simulink model "EPT"  (R2019b)
settings: Solver=FixedStepDiscrete  StartTime=0.0  StopTime=5  FixedStep=0.005  RelTol=1e-3  EnableMultiTasking=on
PreLoadFcn:
  | try, model_open; catch, disp('Error occurred while executing model pre-load callback: model_open.m'); disp('Please assure that the MATLAB working directory is set to the model directory before opening.'); end
InitFcn:
  | try, model_open; catch, end
undefined symbols (not defined in the file or in its folder): Bridge, GCM, H, ln, raptor_get_param_eval, raptor_get_safe_string, raptor_xcp_function
libraries: Raptor_lib x2810, simulink x374, hdlsllib x19
(part 10 of 45)

== system EPT/Foreground_TimeBase_5ms/Oil//Water//Pack Cooling System/AirC1/Delay1 ==
  Condition : Inport
  TimeCount : Inport  Port=2
  Constant10 : Constant
  Constant11 : Constant  Value=0
  Constant8 : Constant  Value=0
  CycleTrigger : Subsystem
  Switch2 : Switch  Threshold=1
  Switch3 : Switch  Threshold=1
  Unit Delay1 : UnitDelay  SampleTime=-1  HasFrameUpgradeWarning=on
  Unit Delay3 : UnitDelay  SampleTime=-1  HasFrameUpgradeWarning=on
  Output : Outport  VectorParamsAs1DForOutWhenUnconnected=off
  wires:
  TimeCount/1 -> CycleTrigger/2(In2)
  Condition/1 -> Switch3/2
  Constant8/1 -> Switch2/1
  CycleTrigger/1(Trigger) -> Switch2/2, Unit Delay3/1
  Constant10/1 -> Switch2/3
  Switch3/1 -> CycleTrigger/1(In1)
  Switch2/1 -> Unit Delay1/1
  Constant11/1 -> Switch3/3
  Unit Delay1/1 -> Switch3/1
  Unit Delay3/1 -> Output/1

== system EPT/Foreground_TimeBase_5ms/Oil//Water//Pack Cooling System/AirC1/Delay2 ==
  Condition : Inport
  TimeCount : Inport  Port=2
  Constant10 : Constant
  Constant11 : Constant  Value=0
  Constant8 : Constant  Value=0
  CycleTrigger : Subsystem
  Switch2 : Switch  Threshold=1
  Switch3 : Switch  Threshold=1
  Unit Delay1 : UnitDelay  SampleTime=-1  HasFrameUpgradeWarning=on
  Unit Delay3 : UnitDelay  SampleTime=-1  HasFrameUpgradeWarning=on
  Output : Outport  VectorParamsAs1DForOutWhenUnconnected=off
  wires:
  TimeCount/1 -> CycleTrigger/2(In2)
  Condition/1 -> Switch3/2
  Constant8/1 -> Switch2/1
  CycleTrigger/1(Trigger) -> Switch2/2, Unit Delay3/1
  Constant10/1 -> Switch2/3
  Switch3/1 -> CycleTrigger/1(In1)
  Switch2/1 -> Unit Delay1/1
  Constant11/1 -> Switch3/3
  Unit Delay1/1 -> Switch3/1
  Unit Delay3/1 -> Output/1

== system EPT/Foreground_TimeBase_5ms/Oil//Water//Pack Cooling System/AirC1/Delay3 ==
  Condition : Inport
  TimeCount : Inport  Port=2
  Constant10 : Constant
  Constant11 : Constant  Value=0
  Constant8 : Constant  Value=0
  CycleTrigger : Subsystem
  Switch2 : Switch  Threshold=1
  Switch3 : Switch  Threshold=1
  Unit Delay1 : UnitDelay  SampleTime=-1  HasFrameUpgradeWarning=on
  Unit Delay3 : UnitDelay  SampleTime=-1  HasFrameUpgradeWarning=on
  Output : Outport  VectorParamsAs1DForOutWhenUnconnected=off
  wires:
  Unit Delay3/1 -> Output/1
  Unit Delay1/1 -> Switch3/1
  Constant11/1 -> Switch3/3
  Switch2/1 -> Unit Delay1/1
  Switch3/1 -> CycleTrigger/1(In1)
  Constant10/1 -> Switch2/3
  CycleTrigger/1(Trigger) -> Unit Delay3/1, Switch2/2
  Constant8/1 -> Switch2/1
  Condition/1 -> Switch3/2
  TimeCount/1 -> CycleTrigger/2(In2)

== system EPT/Foreground_TimeBase_5ms/Oil//Water//Pack Cooling System/AirC1/Delay5 ==
  Condition : Inport
  TimeCount : Inport  Port=2
  Constant10 : Constant
  Constant11 : Constant  Value=0
  Constant8 : Constant  Value=0
  CycleTrigger : Subsystem
  Switch2 : Switch  Threshold=1
  Switch3 : Switch  Threshold=1
  Unit Delay1 : UnitDelay  SampleTime=-1  HasFrameUpgradeWarning=on
  Unit Delay3 : UnitDelay  SampleTime=-1  HasFrameUpgradeWarning=on
  Output : Outport  VectorParamsAs1DForOutWhenUnconnected=off
  wires:
  Unit Delay3/1 -> Output/1
  Unit Delay1/1 -> Switch3/1
  Constant11/1 -> Switch3/3
  Switch2/1 -> Unit Delay1/1
  Switch3/1 -> CycleTrigger/1(In1)
  Constant10/1 -> Switch2/3
  CycleTrigger/1(Trigger) -> Unit Delay3/1, Switch2/2
  Constant8/1 -> Switch2/1
  Condition/1 -> Switch3/2
  TimeCount/1 -> CycleTrigger/2(In2)

== system EPT/Foreground_TimeBase_5ms/Oil//Water//Pack Cooling System/AirC1/Delay6 ==
  Condition : Inport
  TimeCount : Inport  Port=2
  Constant10 : Constant
  Constant11 : Constant  Value=0
  Constant8 : Constant  Value=0
  CycleTrigger : Subsystem
  Switch2 : Switch  Threshold=1
  Switch3 : Switch  Threshold=1
  Unit Delay1 : UnitDelay  SampleTime=-1  HasFrameUpgradeWarning=on
  Unit Delay3 : UnitDelay  SampleTime=-1  HasFrameUpgradeWarning=on
  Output : Outport  VectorParamsAs1DForOutWhenUnconnected=off
  wires:
  Unit Delay3/1 -> Output/1
  Unit Delay1/1 -> Switch3/1
  Constant11/1 -> Switch3/3
  Switch2/1 -> Unit Delay1/1
  Switch3/1 -> CycleTrigger/1(In1)
  Constant10/1 -> Switch2/3
  CycleTrigger/1(Trigger) -> Unit Delay3/1, Switch2/2
  Constant8/1 -> Switch2/1
  Condition/1 -> Switch3/2
  TimeCount/1 -> CycleTrigger/2(In2)

== system EPT/Foreground_TimeBase_5ms/Oil//Water//Pack Cooling System/AirC1/Delay7 ==
  Condition : Inport
  TimeCount : Inport  Port=2
  Constant10 : Constant
  Constant11 : Constant  Value=0
  Constant8 : Constant  Value=0
  CycleTrigger : Subsystem
  Switch2 : Switch  Threshold=1
  Switch3 : Switch  Threshold=1
  Unit Delay1 : UnitDelay  SampleTime=-1  HasFrameUpgradeWarning=on
  Unit Delay3 : UnitDelay  SampleTime=-1  HasFrameUpgradeWarning=on
  Output : Outport  VectorParamsAs1DForOutWhenUnconnected=off
  wires:
  Unit Delay3/1 -> Output/1
  Unit Delay1/1 -> Switch3/1
  Constant11/1 -> Switch3/3
  Switch2/1 -> Unit Delay1/1
  Switch3/1 -> CycleTrigger/1(In1)
  Constant10/1 -> Switch2/3
  CycleTrigger/1(Trigger) -> Unit Delay3/1, Switch2/2
  Constant8/1 -> Switch2/1
  Condition/1 -> Switch3/2
  TimeCount/1 -> CycleTrigger/2(In2)

== system EPT/Foreground_TimeBase_5ms/Oil//Water//Pack Cooling System/AirC1/Latch ==
  Latch : Inport
  Reset : Inport  Port=2
  Switch1 : Switch  Criteria=u2 > Threshold
  Switch3 : Switch  Criteria=u2 > Threshold
  Unit Delay1 : UnitDelay  SampleTime=-1  HasFrameUpgradeWarning=on
  Output : Outport  VectorParamsAs1DForOutWhenUnconnected=off
  wires:
  Unit Delay1/1 -> Switch1/3
  Switch3/1 -> Output/1, Unit Delay1/1
  Reset/1 -> Switch3/2
  Latch/1 -> Switch1/1, Switch1/2
  Switch1/1 -> Switch3/3

== system EPT/Foreground_TimeBase_5ms/Oil//Water//Pack Cooling System/AirC1/Latch1 ==
  Latch : Inport
  Reset : Inport  Port=2
  Switch1 : Switch  Criteria=u2 > Threshold
  Switch3 : Switch  Criteria=u2 > Threshold
  Unit Delay1 : UnitDelay  SampleTime=-1  HasFrameUpgradeWarning=on
  Output : Outport  VectorParamsAs1DForOutWhenUnconnected=off
  wires:
  Unit Delay1/1 -> Switch1/3
  Switch3/1 -> Output/1, Unit Delay1/1
  Reset/1 -> Switch3/2
  Latch/1 -> Switch1/1, Switch1/2
  Switch1/1 -> Switch3/3

== system EPT/Foreground_TimeBase_5ms/Oil//Water//Pack Cooling System/AirC1/Latch2 ==
  Latch : Inport
  Reset : Inport  Port=2
  Switch1 : Switch  Criteria=u2 > Threshold
  Switch3 : Switch  Criteria=u2 > Threshold
  Unit Delay1 : UnitDelay  SampleTime=-1  HasFrameUpgradeWarning=on
  Output : Outport  VectorParamsAs1DForOutWhenUnconnected=off
  wires:
  Switch1/1 -> Switch3/3
  Latch/1 -> Switch1/2, Switch1/1
  Reset/1 -> Switch3/2
  Switch3/1 -> Unit Delay1/1, Output/1
  Unit Delay1/1 -> Switch1/3

== system EPT/Foreground_TimeBase_5ms/Oil//Water//Pack Cooling System/Delay1/CycleTrigger ==
  In1 : Inport
  In2 : Inport  Port=2
  Add : Sum
  Add1 : Sum
  Add2 : Sum  Inputs=+-
  Constant1 : Constant
  Constant2 : Constant  Value=0
  Constant3 : Constant
  Data Type Conversion1 : DataTypeConversion
  Data Type Conversion2 : DataTypeConversion
  Display : Display
  Relational Operator1 : RelationalOperator  OutDataTypeStr=boolean  RndMeth=Simplest
  Saturation : Saturate  UpperLimit=inf  LowerLimit=2
  Scope : Scope
  Scope1 : Scope
  Scope2 : Scope
  Switch : Switch  Threshold=1
  Unit Delay : UnitDelay  SampleTime=-1  HasFrameUpgradeWarning=on
  Unit Delay1 : UnitDelay  SampleTime=-1  HasFrameUpgradeWarning=on
  Trigger : Outport  VectorParamsAs1DForOutWhenUnconnected=off
  wires:
  Saturation/1 -> Add2/1
  Add/1 -> Switch/1
  In1/1 -> Data Type Conversion2/1
  Unit Delay/1 -> Add/1
  Switch/1 -> Relational Operator1/1, Scope1/1, Unit Delay/1
  Add1/1 -> Scope/1, Unit Delay1/1, Display/1
  Unit Delay1/1 -> Add1/1
  Constant1/1 -> Add1/2
  Relational Operator1/1 -> Scope2/1, Trigger/1
  Data Type Conversion1/1 -> Relational Operator1/2
  Constant2/1 -> Switch/3
  Data Type Conversion2/1 -> Add/2, Switch/2
  Add2/1 -> Data Type Conversion1/1
  In2/1 -> Saturation/1
  Constant3/1 -> Add2/2

== system EPT/Foreground_TimeBase_5ms/Oil//Water//Pack Cooling System/Delay2/CycleTrigger ==
  In1 : Inport
  In2 : Inport  Port=2
  Add : Sum
  Add1 : Sum
  Add2 : Sum  Inputs=+-
  Constant1 : Constant
  Constant2 : Constant  Value=0
  Constant3 : Constant
  Data Type Conversion1 : DataTypeConversion
  Data Type Conversion2 : DataTypeConversion
  Display : Display
  Relational Operator1 : RelationalOperator  OutDataTypeStr=boolean  RndMeth=Simplest
  Saturation : Saturate  UpperLimit=inf  LowerLimit=2
  Scope : Scope
  Scope1 : Scope
  Scope2 : Scope
  Switch : Switch  Threshold=1
  Unit Delay : UnitDelay  SampleTime=-1  HasFrameUpgradeWarning=on
  Unit Delay1 : UnitDelay  SampleTime=-1  HasFrameUpgradeWarning=on
  Trigger : Outport  VectorParamsAs1DForOutWhenUnconnected=off
  wires:
  Saturation/1 -> Add2/1
  Add/1 -> Switch/1
  In1/1 -> Data Type Conversion2/1
  Unit Delay/1 -> Add/1
  Switch/1 -> Relational Operator1/1, Scope1/1, Unit Delay/1
  Add1/1 -> Scope/1, Unit Delay1/1, Display/1
  Unit Delay1/1 -> Add1/1
  Constant1/1 -> Add1/2
  Relational Operator1/1 -> Scope2/1, Trigger/1
  Data Type Conversion1/1 -> Relational Operator1/2
  Constant2/1 -> Switch/3
  Data Type Conversion2/1 -> Add/2, Switch/2
  Add2/1 -> Data Type Conversion1/1
  In2/1 -> Saturation/1
  Constant3/1 -> Add2/2

== system EPT/Foreground_TimeBase_5ms/Oil//Water//Pack Cooling System/Delay3/CycleTrigger ==
  In1 : Inport
  In2 : Inport  Port=2
  Add : Sum
  Add1 : Sum
  Add2 : Sum  Inputs=+-
  Constant1 : Constant
  Constant2 : Constant  Value=0
  Constant3 : Constant
  Data Type Conversion1 : DataTypeConversion
  Data Type Conversion2 : DataTypeConversion
  Display : Display
  Relational Operator1 : RelationalOperator  OutDataTypeStr=boolean  RndMeth=Simplest
  Saturation : Saturate  UpperLimit=inf  LowerLimit=2
  Scope : Scope
  Scope1 : Scope
  Scope2 : Scope
  Switch : Switch  Threshold=1
  Unit Delay : UnitDelay  SampleTime=-1  HasFrameUpgradeWarning=on
  Unit Delay1 : UnitDelay  SampleTime=-1  HasFrameUpgradeWarning=on
  Trigger : Outport  VectorParamsAs1DForOutWhenUnconnected=off
  wires:
  Constant3/1 -> Add2/2
  In2/1 -> Saturation/1
  Add2/1 -> Data Type Conversion1/1
  Data Type Conversion2/1 -> Switch/2, Add/2
  Constant2/1 -> Switch/3
  Data Type Conversion1/1 -> Relational Operator1/2
  Relational Operator1/1 -> Trigger/1, Scope2/1
  Constant1/1 -> Add1/2
  Unit Delay1/1 -> Add1/1
  Add1/1 -> Display/1, Unit Delay1/1, Scope/1
  Switch/1 -> Unit Delay/1, Scope1/1, Relational Operator1/1
  Unit Delay/1 -> Add/1
  In1/1 -> Data Type Conversion2/1
  Add/1 -> Switch/1
  Saturation/1 -> Add2/1

== system EPT/Foreground_TimeBase_5ms/Oil//Water//Pack Cooling System/Delay5/CycleTrigger ==
  In1 : Inport
  In2 : Inport  Port=2
  Add : Sum
  Add1 : Sum
  Add2 : Sum  Inputs=+-
  Constant1 : Constant
  Constant2 : Constant  Value=0
  Constant3 : Constant
  Data Type Conversion1 : DataTypeConversion
  Data Type Conversion2 : DataTypeConversion
  Display : Display
  Relational Operator1 : RelationalOperator  OutDataTypeStr=boolean  RndMeth=Simplest
  Saturation : Saturate  UpperLimit=inf  LowerLimit=2
  Scope : Scope
  Scope1 : Scope
  Scope2 : Scope
  Switch : Switch  Threshold=1
  Unit Delay : UnitDelay  SampleTime=-1  HasFrameUpgradeWarning=on
  Unit Delay1 : UnitDelay  SampleTime=-1  HasFrameUpgradeWarning=on
  Trigger : Outport  VectorParamsAs1DForOutWhenUnconnected=off
  wires:
  Constant3/1 -> Add2/2
  In2/1 -> Saturation/1
  Add2/1 -> Data Type Conversion1/1
  Data Type Conversion2/1 -> Switch/2, Add/2
  Constant2/1 -> Switch/3
  Data Type Conversion1/1 -> Relational Operator1/2
  Relational Operator1/1 -> Trigger/1, Scope2/1
  Constant1/1 -> Add1/2
  Unit Delay1/1 -> Add1/1
  Add1/1 -> Display/1, Unit Delay1/1, Scope/1
  Switch/1 -> Unit Delay/1, Scope1/1, Relational Operator1/1
  Unit Delay/1 -> Add/1
  In1/1 -> Data Type Conversion2/1
  Add/1 -> Switch/1
  Saturation/1 -> Add2/1

== system EPT/Foreground_TimeBase_5ms/Oil//Water//Pack Cooling System/Delay6/CycleTrigger ==
  In1 : Inport
  In2 : Inport  Port=2
  Add : Sum
  Add1 : Sum
  Add2 : Sum  Inputs=+-
  Constant1 : Constant
  Constant2 : Constant  Value=0
  Constant3 : Constant
  Data Type Conversion1 : DataTypeConversion
  Data Type Conversion2 : DataTypeConversion
  Display : Display
  Relational Operator1 : RelationalOperator  OutDataTypeStr=boolean  RndMeth=Simplest
  Saturation : Saturate  UpperLimit=inf  LowerLimit=2
  Scope : Scope
  Scope1 : Scope
  Scope2 : Scope
  Switch : Switch  Threshold=1
  Unit Delay : UnitDelay  SampleTime=-1  HasFrameUpgradeWarning=on
  Unit Delay1 : UnitDelay  SampleTime=-1  HasFrameUpgradeWarning=on
  Trigger : Outport  VectorParamsAs1DForOutWhenUnconnected=off
  wires:
  Constant3/1 -> Add2/2
  In2/1 -> Saturation/1
  Add2/1 -> Data Type Conversion1/1
  Data Type Conversion2/1 -> Switch/2, Add/2
  Constant2/1 -> Switch/3
  Data Type Conversion1/1 -> Relational Operator1/2
  Relational Operator1/1 -> Trigger/1, Scope2/1
  Constant1/1 -> Add1/2
  Unit Delay1/1 -> Add1/1
  Add1/1 -> Display/1, Unit Delay1/1, Scope/1
  Switch/1 -> Unit Delay/1, Scope1/1, Relational Operator1/1
  Unit Delay/1 -> Add/1
  In1/1 -> Data Type Conversion2/1
  Add/1 -> Switch/1
  Saturation/1 -> Add2/1

== system EPT/Foreground_TimeBase_5ms/Oil//Water//Pack Cooling System/Delay7/CycleTrigger ==
  In1 : Inport
  In2 : Inport  Port=2
  Add : Sum
  Add1 : Sum
  Add2 : Sum  Inputs=+-
  Constant1 : Constant
  Constant2 : Constant  Value=0
  Constant3 : Constant
  Data Type Conversion1 : DataTypeConversion
  Data Type Conversion2 : DataTypeConversion
  Display : Display
  Relational Operator1 : RelationalOperator  OutDataTypeStr=boolean  RndMeth=Simplest
  Saturation : Saturate  UpperLimit=inf  LowerLimit=2
  Scope : Scope
  Scope1 : Scope
  Scope2 : Scope
  Switch : Switch  Threshold=1
  Unit Delay : UnitDelay  SampleTime=-1  HasFrameUpgradeWarning=on
  Unit Delay1 : UnitDelay  SampleTime=-1  HasFrameUpgradeWarning=on
  Trigger : Outport  VectorParamsAs1DForOutWhenUnconnected=off
  wires:
  Constant3/1 -> Add2/2
  In2/1 -> Saturation/1
  Add2/1 -> Data Type Conversion1/1
  Data Type Conversion2/1 -> Switch/2, Add/2
  Constant2/1 -> Switch/3
  Data Type Conversion1/1 -> Relational Operator1/2
  Relational Operator1/1 -> Trigger/1, Scope2/1
  Constant1/1 -> Add1/2
  Unit Delay1/1 -> Add1/1
  Add1/1 -> Display/1, Unit Delay1/1, Scope/1
  Switch/1 -> Unit Delay/1, Scope1/1, Relational Operator1/1
  Unit Delay/1 -> Add/1
  In1/1 -> Data Type Conversion2/1
  Add/1 -> Switch/1
  Saturation/1 -> Add2/1

== system EPT/Foreground_TimeBase_5ms/System Initial/Delay1/CycleTrigger ==
  In1 : Inport
  In2 : Inport  Port=2
  Add : Sum
  Add1 : Sum
  Add2 : Sum  Inputs=+-
  Constant1 : Constant
  Constant2 : Constant  Value=0
  Constant3 : Constant
  Data Type Conversion1 : DataTypeConversion
  Data Type Conversion2 : DataTypeConversion
  Display : Display
  Relational Operator1 : RelationalOperator  OutDataTypeStr=boolean  RndMeth=Simplest
  Saturation : Saturate  UpperLimit=inf  LowerLimit=2
  Scope : Scope
  Scope1 : Scope
  Scope2 : Scope
  Switch : Switch  Threshold=1
  Unit Delay : UnitDelay  SampleTime=-1  HasFrameUpgradeWarning=on
  Unit Delay1 : UnitDelay  SampleTime=-1  HasFrameUpgradeWarning=on
  Trigger : Outport  VectorParamsAs1DForOutWhenUnconnected=off
  wires:
  Saturation/1 -> Add2/1
  Add/1 -> Switch/1
  In1/1 -> Data Type Conversion2/1
  Unit Delay/1 -> Add/1
  Switch/1 -> Relational Operator1/1, Scope1/1, Unit Delay/1
  Add1/1 -> Scope/1, Unit Delay1/1, Display/1
  Unit Delay1/1 -> Add1/1
  Constant1/1 -> Add1/2
  Relational Operator1/1 -> Scope2/1, Trigger/1
  Data Type Conversion1/1 -> Relational Operator1/2
  Constant2/1 -> Switch/3
  Data Type Conversion2/1 -> Add/2, Switch/2
  Add2/1 -> Data Type Conversion1/1
  In2/1 -> Saturation/1
  Constant3/1 -> Add2/2

== system EPT/Foreground_TimeBase_5ms/System Initial/Shutdown_Event_Related/Relaybox_Related ==
  Init : Inport
  Data Type Conversion3 : DataTypeConversion
  NOT : Logic  Operator=NOT  IconShape=distinctive  AllPortsSameDT=off  OutDataTypeStr=boolean
  raptor_data_write1 : Raptor_lib/Data Storage/raptor_data_write  dataName='Relay_CHG_OBC'  dataShape=Scalar  idxSource=Input Port  idxRow=1  idxCol=1
      settings: SourceProductName=Raptor
  raptor_data_write19 : Raptor_lib/Data Storage/raptor_data_write  dataName='Relay_BMS_OBU'  dataShape=Scalar  idxSource=Input Port  idxRow=1  idxCol=1
      settings: SourceProductName=Raptor
  raptor_data_write2 : Raptor_lib/Data Storage/raptor_data_write  dataName='Cmd_DC_Control'  dataShape=Scalar  idxSource=Input Port  idxRow=1  idxCol=1
      settings: SourceProductName=Raptor
  raptor_data_write20 : Raptor_lib/Data Storage/raptor_data_write  dataName='Relay_BMS_SWU'  dataShape=Scalar  idxSource=Input Port  idxRow=1  idxCol=1
      settings: SourceProductName=Raptor
  raptor_data_write21 : Raptor_lib/Data Storage/raptor_data_write  dataName='Relay_MCU'  dataShape=Scalar  idxSource=Input Port  idxRow=1  idxCol=1
      settings: SourceProductName=Raptor
  raptor_data_write27 : Raptor_lib/Data Storage/raptor_data_write  dataName='Relay_DCDC_12V'  dataShape=Scalar  idxSource=Input Port  idxRow=1  idxCol=1
      settings: SourceProductName=Raptor
  wires:
  NOT/1 -> Data Type Conversion3/1
  Data Type Conversion3/1 -> raptor_data_write2/1
  Init/1 -> raptor_data_write27/1, raptor_data_write19/1, raptor_data_write20/1, raptor_data_write21/1, raptor_data_write1/1, NOT/1

== system EPT/Foreground_TimeBase_5ms/System Setup/Dyno_Test /Dyno Test ==
  note: 'manual_or_automatic':
      | 0=Manual
      | 1=Automatic Inc
  note: 'Enable':
      | 0=Enable Function
      | 1=Disable Function
  note: 'Torque_Max':
  note: 'Target_Torque_Manual':
  note: 'Torque_Inc_unit':
  Bitwise Operator : simulink/Logic and Bit Operations/Bitwise Operator  logicop=XOR  UseBitMask=off  NumInputPorts=2  BitMask=bin2dec('11011001')  BitMaskRealWorld=Stored Integer
  Detect Change : simulink/Logic and Bit Operations/Detect Change  vinit=10  OutDataTypeStr=boolean
  Detect Change1 : simulink/Logic and Bit Operations/Detect Change  vinit=10  OutDataTypeStr=boolean
  Latch : Subsystem
  Logical Operator1 : Logic  Operator=OR  AllPortsSameDT=off  OutDataTypeStr=boolean
  Logical Operator2 : Logic  AllPortsSameDT=off  OutDataTypeStr=boolean
  Logical Operator3 : Logic  AllPortsSameDT=off  OutDataTypeStr=boolean
  Logical Operator4 : Logic  AllPortsSameDT=off  OutDataTypeStr=boolean
  Logical Operator5 : Logic  Operator=OR  AllPortsSameDT=off  OutDataTypeStr=boolean
  MCU Tq MAP_Inc : Subsystem
  MCU Tq MAP_Manual : Subsystem
  NOT : Logic  Operator=NOT  IconShape=distinctive  AllPortsSameDT=off  OutDataTypeStr=boolean
  Relational Operator : RelationalOperator  Operator===  OutDataTypeStr=boolean  RndMeth=Simplest
  Relational Operator1 : RelationalOperator  Operator===  OutDataTypeStr=boolean  RndMeth=Simplest
  Switch2 : Switch  Criteria=u2 > Threshold
  Switch4 : Switch  Criteria=u2 > Threshold
  raptor_adjustment : Raptor_lib/Data Storage/raptor_adjustment  paramName='Target_Torque_Manual'  nameSource=Parameter  initValue=0  dataType=double  storage=Calibration  calDispType=Number  calEnum={'False', 'True'}  calGain=1.0  calOffset=0.0  calMax=150  calMin=-150  calFormat='-1'  calUnit=''  calHelp=''  calAccess=1  calFunction=raptor_xcp_function(gcb)  calDispHeaders=off  calColHeaders={'Col1' 'Col2' 'Col3'}  calRowHeaders={'Row1' 'Row2' 'Row3'}
      settings: SourceProductName=Raptor
  raptor_adjustment1 : Raptor_lib/Data Storage/raptor_adjustment  paramName='Enable'  nameSource=Parameter  initValue=0  dataType=boolean  storage=Calibration  calDispType=Number  calEnum={'False', 'True'}  calGain=1.0  calOffset=0.0  calMax=inf  calMin=-inf  calFormat='-1'  calUnit=''  calHelp=''  calAccess=1  calFunction=raptor_xcp_function(gcb)  calDispHeaders=off  calColHeaders={'Col1' 'Col2' 'Col3'}  calRowHeaders={'Row1' 'Row2' 'Row3'}
      settings: SourceProductName=Raptor
  raptor_adjustment2 : Raptor_lib/Data Storage/raptor_adjustment  paramName='manual_or_automatic'  nameSource=Parameter  initValue=0  dataType=boolean  storage=Calibration  calDispType=Number  calEnum={'False', 'True'}  calGain=1.0  calOffset=0.0  calMax=inf  calMin=-inf  calFormat='-1'  calUnit=''  calHelp=''  calAccess=1  calFunction=raptor_xcp_function(gcb)  calDispHeaders=off  calColHeaders={'Col1' 'Col2' 'Col3'}  calRowHeaders={'Row1' 'Row2' 'Row3'}
      settings: SourceProductName=Raptor
  raptor_adjustment3 : Raptor_lib/Data Storage/raptor_adjustment  paramName='Torque_Max'  nameSource=Parameter  initValue=100  dataType=double  storage=Calibration  calDispType=Number  calEnum={'False', 'True'}  calGain=1.0  calOffset=0.0  calMax=150  calMin=-150  calFormat='-1'  calUnit=''  calHelp=''  calAccess=1  calFunction=raptor_xcp_function(gcb)  calDispHeaders=off  calColHeaders={'Col1' 'Col2' 'Col3'}  calRowHeaders={'Row1' 'Row2' 'Row3'}
      settings: SourceProductName=Raptor
  raptor_adjustment4 : Raptor_lib/Data Storage/raptor_adjustment  paramName='Torque_Inc_unit'  nameSource=Parameter  initValue=0  dataType=double  storage=Calibration  calDispType=Number  calEnum={'False', 'True'}  calGain=1.0  calOffset=0.0  calMax=inf  calMin=-inf  calFormat='-1'  calUnit=''  calHelp=''  calAccess=1  calFunction=raptor_xcp_function(gcb)  calDispHeaders=off  calColHeaders={'Col1' 'Col2' 'Col3'}  calRowHeaders={'Row1' 'Row2' 'Row3'}
      settings: SourceProductName=Raptor
  raptor_adjustment5 : Raptor_lib/Data Storage/raptor_adjustment  paramName='Forward_Switch'  nameSource=Parameter  initValue=0  dataType=boolean  storage=Calibration  calDispType=Number  calEnum={'False', 'True'}  calGain=1.0  calOffset=0.0  calMax=inf  calMin=-inf  calFormat='-1'  calUnit=''  calHelp=''  calAccess=1  calFunction=raptor_xcp_function(gcb)  calDispHeaders=off  calColHeaders={'Col1' 'Col2' 'Col3'}  calRowHeaders={'Row1' 'Row2' 'Row3'}
      settings: SourceProductName=Raptor
  raptor_adjustment6 : Raptor_lib/Data Storage/raptor_adjustment  paramName='Reverse_Switch'  nameSource=Parameter  initValue=0  dataType=boolean  storage=Calibration  calDispType=Number  calEnum={'False', 'True'}  calGain=1.0  calOffset=0.0  calMax=inf  calMin=-inf  calFormat='-1'  calUnit=''  calHelp=''  calAccess=1  calFunction=raptor_xcp_function(gcb)  calDispHeaders=off  calColHeaders={'Col1' 'Col2' 'Col3'}  calRowHeaders={'Row1' 'Row2' 'Row3'}
      settings: SourceProductName=Raptor
  Command_Tq : Outport  VectorParamsAs1DForOutWhenUnconnected=off
  Flag : Outport  Port=2  VectorParamsAs1DForOutWhenUnconnected=off
  wires:
  raptor_adjustment3/1 -> MCU Tq MAP_Manual/2(Tq_Max), MCU Tq MAP_Inc/2(Tq_Max)
  NOT/1 -> Logical Operator4/2, Switch2/2
  raptor_adjustment2/1 -> Detect Change/1, NOT/1, Logical Operator2/2
  raptor_adjustment1/1 -> MCU Tq MAP_Manual/1(Enable), Detect Change1/1, MCU Tq MAP_Inc/1(Enable)
  MCU Tq MAP_Inc/1(Command_Tq) -> Switch2/3
  MCU Tq MAP_Manual/1(Command_Tq) -> Switch2/1
  Switch4/1 -> Command_Tq/1
  Switch2/1 -> Switch4/1
  MCU Tq MAP_Inc/2(Flag) -> Flag/1
  raptor_adjustment5/1 -> Bitwise Operator/1
  raptor_adjustment6/1 -> Bitwise Operator/2
  Latch/1(Output) -> Logical Operator3/1
  Bitwise Operator/1 -> Logical Operator3/2
  Logical Operator3/1 -> Switch4/2
  Logical Operator1/1 -> Latch/1(Latch)
  Logical Operator4/1 -> Logical Operator1/1
  Logical Operator2/1 -> Logical Operator1/2
  Relational Operator/1 -> Logical Operator4/1
  Relational Operator1/1 -> Logical Operator2/1
  raptor_adjustment/1 -> Relational Operator/2, MCU Tq MAP_Manual/3(Target_Torque_Manual)
  raptor_adjustment4/1 -> Relational Operator1/2, MCU Tq MAP_Inc/3(Torque_Inc_unit)
  Logical Operator5/1 -> Latch/2(Reset)
  Detect Change/1 -> Logical Operator5/1
  Detect Change1/1 -> Logical Operator5/2

== system EPT/Foreground_TimeBase_5ms/System Setup/HV_Setup()/CHG_Mode ==
  note: Notes :
      | - PreCHG has been completed and (Drive Mode is OFF&&CHG Mode is ON),allowing CHG Mode.
      | - CHG Mode is OFF,Disable CHG Mode
  CHG Full Flag : Subsystem  Commented=on
  CHG_Mode_Function : Subsystem
  Constant : Constant  Value=0  OutDataTypeStr=boolean
  Delay : Delay
  Delay1 : Subsystem
  Disable_CHG_Mode_Function : Subsystem
  Latch1 : Subsystem
  Logical Operator : Logic  Inputs=5  AllPortsSameDT=off  OutDataTypeStr=boolean
  Logical Operator1 : Logic  Inputs=3  AllPortsSameDT=off  OutDataTypeStr=boolean
  Logical Operator3 : Logic  Operator=OR  Inputs=4  AllPortsSameDT=off  OutDataTypeStr=boolean
  NOT{,1..3} (4 alike) : Logic  Operator=NOT  IconShape=distinctive  AllPortsSameDT=off  OutDataTypeStr=boolean
  Switch : Switch  Criteria=u2 > Threshold
  raptor_adjustment1 : Raptor_lib/Data Storage/raptor_adjustment  paramName='Delay_EVSE_EOC_EN'  nameSource=Parameter  initValue=100  dataType=double  storage=Calibration  calDispType=Number  calEnum={'False', 'True'}  calGain=1.0  calOffset=0.0  calMax=inf  calMin=-inf  calFormat='-1'  calUnit=''  calHelp=''  calAccess=1  calFunction=raptor_xcp_function(gcb)  calDispHeaders=off  calColHeaders={'Col1' 'Col2' 'Col3'}  calRowHeaders={'Row1' 'Row2' 'Row3'}
      settings: SourceProductName=Raptor
  raptor_data_read1 : Raptor_lib/Data Storage/raptor_data_read  dataName='Flag_HV_Drive_Relay_On'  dataShape=Scalar  idxSource=Input  idxRow=1  idxCol=1
      settings: SourceProductName=Raptor
  raptor_data_read10 : Raptor_lib/Data Storage/raptor_data_read  dataName='K35_CHG_Request'  dataShape=Scalar  idxSource=Input  idxRow=1  idxCol=1
      settings: SourceProductName=Raptor
  raptor_data_read11 : Raptor_lib/Data Storage/raptor_data_read  dataName='Flag_CHG_Mode'  dataShape=Scalar  idxSource=Input  idxRow=1  idxCol=1
      settings: SourceProductName=Raptor
  raptor_data_read14 : Raptor_lib/Data Storage/raptor_data_read  dataName='Fault_Reset_Trigger'  dataShape=Scalar  idxSource=Input  idxRow=1  idxCol=1
      settings: SourceProductName=Raptor
  raptor_data_read2 : Raptor_lib/Data Storage/raptor_data_read  dataName='EPT_EW_STA'  dataShape=Scalar  idxSource=Input  idxRow=1  idxCol=1
      settings: SourceProductName=Raptor
  raptor_data_read3 : Raptor_lib/Data Storage/raptor_data_read  dataName='Flag_Drive_Mode'  dataShape=Scalar  idxSource=Input  idxRow=1  idxCol=1
      settings: SourceProductName=Raptor
  raptor_data_read4 : Raptor_lib/Data Storage/raptor_data_read  dataName='Flag_CHG_Mode'  dataShape=Scalar  idxSource=Input  idxRow=1  idxCol=1
      settings: SourceProductName=Raptor
  raptor_data_read5 : Raptor_lib/Data Storage/raptor_data_read  dataName='EPT_EW_STA'  dataShape=Scalar  idxSource=Input  idxRow=1  idxCol=1
      settings: SourceProductName=Raptor
  raptor_data_read6 : Raptor_lib/Data Storage/raptor_data_read  dataName='HV_Off'  dataShape=Scalar  idxSource=Input  idxRow=1  idxCol=1
      settings: SourceProductName=Raptor
  raptor_data_read7 : Raptor_lib/Data Storage/raptor_data_read  dataName='HV_Off'  dataShape=Scalar  idxSource=Input  idxRow=1  idxCol=1
      settings: SourceProductName=Raptor
  raptor_data_read8 : Raptor_lib/Data Storage/raptor_data_read  dataName='EVSE_STATUS_E'  dataShape=Scalar  idxSource=Input  idxRow=1  idxCol=1
      settings: SourceProductName=Raptor
  raptor_data_read9 : Raptor_lib/Data Storage/raptor_data_read  dataName='EVSE_STATUS_F'  dataShape=Scalar  idxSource=Input  idxRow=1  idxCol=1
      settings: SourceProductName=Raptor
  raptor_data_write1 : Raptor_lib/Data Storage/raptor_data_write  dataName='A24_EOC_Enable'  dataShape=Scalar  idxSource=Input Port  idxRow=1  idxCol=1
      settings: SourceProductName=Raptor
  raptor_data_write4 : Raptor_lib/Data Storage/raptor_data_write  dataName='EPT_CHG_REQ'  dataShape=Scalar  idxSource=Input Port  idxRow=1  idxCol=1
      settings: SourceProductName=Raptor
  wires:
  raptor_data_read3/1 -> NOT1/1
  NOT1/1 -> Logical Operator/2
  Logical Operator/1 -> CHG_Mode_Function/Enable, NOT/1
  raptor_data_read4/1 -> Logical Operator/1
  NOT2/1 -> Logical Operator/4
  raptor_data_read1/1 -> Logical Operator/3
  raptor_data_read2/1 -> NOT2/1
  raptor_data_read6/1 -> NOT3/1
  NOT3/1 -> Logical Operator/5
  NOT/1 -> Disable_CHG_Mode_Function/Enable
  raptor_data_read7/1 -> Logical Operator3/4
  raptor_data_read8/1 -> Logical Operator3/1
  raptor_data_read9/1 -> Logical Operator3/2
  raptor_data_read5/1 -> Logical Operator3/3
  raptor_data_read14/1 -> Latch1/2(Reset)
  raptor_data_read10/1 -> Switch/3, Logical Operator1/1
  Switch/1 -> Delay/1
  raptor_data_read11/1 -> Logical Operator1/3
  Delay1/1(Output) -> Latch1/1(Latch)
  raptor_adjustment1/1 -> Delay1/2(TimeCount)
  Logical Operator1/1 -> Delay1/1(Condition)
  Latch1/1(Output) -> Switch/2, raptor_data_write1/1
  Logical Operator3/1 -> Logical Operator1/2
  Delay/1 -> raptor_data_write4/1
  Constant/1 -> Switch/1

== system EPT/Foreground_TimeBase_5ms/System Setup/HV_Setup()/Delay ==
  Condition : Inport
  TimeCount : Inport  Port=2
  Constant10 : Constant
  Constant11 : Constant  Value=0
  Constant8 : Constant  Value=0
  CycleTrigger : Subsystem
  Switch2 : Switch  Threshold=1
  Switch3 : Switch  Threshold=1
  Unit Delay1 : UnitDelay  SampleTime=-1  HasFrameUpgradeWarning=on
  Unit Delay3 : UnitDelay  SampleTime=-1  HasFrameUpgradeWarning=on
  Output : Outport  VectorParamsAs1DForOutWhenUnconnected=off
  wires:
  TimeCount/1 -> CycleTrigger/2(In2)
  Condition/1 -> Switch3/2
  Constant8/1 -> Switch2/1
  CycleTrigger/1(Trigger) -> Switch2/2, Unit Delay3/1
  Constant10/1 -> Switch2/3
  Switch3/1 -> CycleTrigger/1(In1)
  Switch2/1 -> Unit Delay1/1
  Constant11/1 -> Switch3/3
  Unit Delay1/1 -> Switch3/1
  Unit Delay3/1 -> Output/1

== system EPT/Foreground_TimeBase_5ms/System Setup/HV_Setup()/Drive_Mode ==
  note: Notes :
      | - PreCHG has been completed and (Drive Mode is ON&&CHG Mode is OFF),allowing Drive Mode.
      | - Drive Mode is OFF,Disable Drive Mode
  Disable_Drive_Mode : Subsystem
  Drive_Mode_Function : Subsystem
  Logical Operator : Logic  Inputs=5  AllPortsSameDT=off  OutDataTypeStr=boolean
  NOT{,2..4} (4 alike) : Logic  Operator=NOT  IconShape=distinctive  AllPortsSameDT=off  OutDataTypeStr=boolean
  raptor_data_read1 : Raptor_lib/Data Storage/raptor_data_read  dataName='Flag_HV_Drive_Relay_On'  dataShape=Scalar  idxSource=Input  idxRow=1  idxCol=1
      settings: SourceProductName=Raptor
  raptor_data_read2 : Raptor_lib/Data Storage/raptor_data_read  dataName='EPT_EW_STA'  dataShape=Scalar  idxSource=Input  idxRow=1  idxCol=1
      settings: SourceProductName=Raptor
  raptor_data_read3 : Raptor_lib/Data Storage/raptor_data_read  dataName='Flag_Drive_Mode'  dataShape=Scalar  idxSource=Input  idxRow=1  idxCol=1
      settings: SourceProductName=Raptor
  raptor_data_read4 : Raptor_lib/Data Storage/raptor_data_read  dataName='Flag_CHG_Mode'  dataShape=Scalar  idxSource=Input  idxRow=1  idxCol=1
      settings: SourceProductName=Raptor
  raptor_data_read6 : Raptor_lib/Data Storage/raptor_data_read  dataName='HV_Off'  dataShape=Scalar  idxSource=Input  idxRow=1  idxCol=1
      settings: SourceProductName=Raptor
  wires:
  raptor_data_read1/1 -> Logical Operator/3
  raptor_data_read6/1 -> NOT3/1
  raptor_data_read4/1 -> NOT4/1
  raptor_data_read2/1 -> NOT2/1
  NOT3/1 -> Logical Operator/5
  NOT2/1 -> Logical Operator/4
  raptor_data_read3/1 -> Logical Operator/2
  NOT4/1 -> Logical Operator/1
  Logical Operator/1 -> Drive_Mode_Function/Enable, NOT/1
  NOT/1 -> Disable_Drive_Mode/Enable

== system EPT/Foreground_TimeBase_5ms/System Setup/HV_Setup()/Latch ==
  Latch : Inport
  Reset : Inport  Port=2
  Switch1 : Switch  Criteria=u2 > Threshold
  Switch3 : Switch  Criteria=u2 > Threshold
  Unit Delay1 : UnitDelay  SampleTime=-1  HasFrameUpgradeWarning=on
  Output : Outport  VectorParamsAs1DForOutWhenUnconnected=off
  wires:
  Switch1/1 -> Switch3/3
  Latch/1 -> Switch1/2, Switch1/1
  Reset/1 -> Switch3/2
  Switch3/1 -> Unit Delay1/1, Output/1
  Unit Delay1/1 -> Switch1/3

== system EPT/Foreground_TimeBase_5ms/System Setup/HV_Setup()/PreCharge_Arbitration ==
  HV_BPOBU_Voltage : Inport
  HV_Bus_Voltage : Inport  Port=2
  Res : Inport  Port=3
  Cap : Inport  Port=4
  Abs : Abs
  Constant2 : Constant  Value=100
  Constant3 : Constant  Value=10
  Constant4 : Constant  Value=10
  Constant6 : Constant  Value=0
  Constant8 : Constant  Value=0.005
  Constant9 : Constant  Value=6
  Delay : Delay  DelayLengthSource=Input port  DelayLength=1  InitialCondition=0
      settings: InputPortMap=u0,p1
  Divide1 : Product  Inputs=**
  Divide2 : Product  Inputs=**/
  Divide3 : Product  Inputs=*/
  Logical Operator : Logic  Inputs=3  AllPortsSameDT=off  OutDataTypeStr=boolean
  Relational Operator : RelationalOperator  Operator=<=  OutDataTypeStr=boolean  RndMeth=Simplest
  Relational Operator1 : RelationalOperator  Operator=<=  OutDataTypeStr=boolean  RndMeth=Simplest
  Relational Operator2 : RelationalOperator  Operator=<=  OutDataTypeStr=boolean  RndMeth=Simplest
  Relational Operator3 : RelationalOperator  OutDataTypeStr=boolean  RndMeth=Simplest
  Slope_Offset : Subsystem
  Subtract : Sum  Inputs=+-
  Subtract1 : Sum  Inputs=+-
  Switch : Switch  Threshold=1
  PreCHG_Arbitration : Outport  VectorParamsAs1DForOutWhenUnconnected=off
  wires:
  Abs/1 -> Relational Operator1/1, Divide2/1
  Constant4/1 -> Relational Operator1/2
  Constant2/1 -> Divide2/2
  HV_Bus_Voltage/1 -> Slope_Offset/3(Vbatt), Subtract/2, Divide2/3
  Constant3/1 -> Relational Operator/2
  Subtract/1 -> Abs/1
  Divide2/1 -> Relational Operator/1
  Res/1 -> Slope_Offset/1(R_ohm)
  Cap/1 -> Slope_Offset/2(C_uF)
  Delay/1 -> Subtract1/2
  Constant9/1 -> Divide1/1, Delay/2
  Constant8/1 -> Divide1/2
  Subtract1/1 -> Divide3/1
  Divide1/1 -> Divide3/2
  Slope_Offset/1(Slope_Ref) -> Relational Operator2/2
  Divide3/1 -> Switch/1, Relational Operator3/1
  Relational Operator3/1 -> Switch/2
  Constant6/1 -> Relational Operator3/2
  Switch/1 -> Relational Operator2/1
  HV_BPOBU_Voltage/1 -> Delay/1, Subtract1/1, Subtract/1
  Relational Operator1/1 -> Logical Operator/1
  Relational Operator/1 -> Logical Operator/2
  Relational Operator2/1 -> Logical Operator/3
  Logical Operator/1 -> PreCHG_Arbitration/1

== system EPT/Foreground_TimeBase_5ms/System Setup/HV_Setup()/Subsystem ==
  Mode : Inport
  EPT_EW_STAT : Inport  Port=2
  HV_Off : Inport  Port=3
  Constant3 : Constant  Value=25
  Constant4 : Constant  Value=25
  Delay1 : Subsystem
  Delay2 : Subsystem
  Latch1 : Subsystem
  Logical Operator2 : Logic  Operator=OR  Inputs=3  AllPortsSameDT=off  OutDataTypeStr=boolean
  NOT4 : Logic  Operator=NOT  IconShape=distinctive  AllPortsSameDT=off  OutDataTypeStr=boolean
  HV_On : Outport
  wires:
  NOT4/1 -> Logical Operator2/1
  Delay1/1(Output) -> Latch1/1(Latch)
  EPT_EW_STAT/1 -> Logical Operator2/2
  Constant3/1 -> Delay1/2(TimeCount)
  Latch1/1(Output) -> HV_On/1
  Delay2/1(Output) -> Latch1/2(Reset)
  Mode/1 -> Delay1/1(Condition), NOT4/1
  Constant4/1 -> Delay2/2(TimeCount)
  Logical Operator2/1 -> Delay2/1(Condition)
  HV_Off/1 -> Logical Operator2/3

== system EPT/Foreground_TimeBase_5ms/System Setup/Unit_Setup()/Delay ==
  Condition : Inport
  TimeCount : Inport  Port=2
  Constant10 : Constant
  Constant11 : Constant  Value=0
  Constant8 : Constant  Value=0
  CycleTrigger : Subsystem
  Switch2 : Switch  Threshold=1
  Switch3 : Switch  Threshold=1
  Unit Delay1 : UnitDelay  SampleTime=-1  HasFrameUpgradeWarning=on
  Unit Delay3 : UnitDelay  SampleTime=-1  HasFrameUpgradeWarning=on
  Output : Outport  VectorParamsAs1DForOutWhenUnconnected=off
  wires:
  Unit Delay3/1 -> Output/1
  Unit Delay1/1 -> Switch3/1
  Constant11/1 -> Switch3/3
  Switch2/1 -> Unit Delay1/1
  Switch3/1 -> CycleTrigger/1(In1)
  Constant10/1 -> Switch2/3
  CycleTrigger/1(Trigger) -> Unit Delay3/1, Switch2/2
  Constant8/1 -> Switch2/1
  Condition/1 -> Switch3/2
  TimeCount/1 -> CycleTrigger/2(In2)

== system EPT/Foreground_TimeBase_5ms/System Setup/Unit_Setup()/Delay1 ==
  Condition : Inport
  TimeCount : Inport  Port=2
  Constant10 : Constant
  Constant11 : Constant  Value=0
  Constant8 : Constant  Value=0
  CycleTrigger : Subsystem
  Switch2 : Switch  Threshold=1
  Switch3 : Switch  Threshold=1
  Unit Delay1 : UnitDelay  SampleTime=-1  HasFrameUpgradeWarning=on
  Unit Delay3 : UnitDelay  SampleTime=-1  HasFrameUpgradeWarning=on
  Output : Outport  VectorParamsAs1DForOutWhenUnconnected=off
  wires:
  Unit Delay3/1 -> Output/1
  Unit Delay1/1 -> Switch3/1
  Constant11/1 -> Switch3/3
  Switch2/1 -> Unit Delay1/1
  Switch3/1 -> CycleTrigger/1(In1)
  Constant10/1 -> Switch2/3
  CycleTrigger/1(Trigger) -> Unit Delay3/1, Switch2/2
  Constant8/1 -> Switch2/1
  Condition/1 -> Switch3/2
  TimeCount/1 -> CycleTrigger/2(In2)

== system EPT/Foreground_TimeBase_5ms/System Setup/Unit_Setup()/Delay2 ==
  Condition : Inport
  TimeCount : Inport  Port=2
  Constant10 : Constant
  Constant11 : Constant  Value=0
  Constant8 : Constant  Value=0
  CycleTrigger : Subsystem
  Switch2 : Switch  Threshold=1
  Switch3 : Switch  Threshold=1
  Unit Delay1 : UnitDelay  SampleTime=-1  HasFrameUpgradeWarning=on
  Unit Delay3 : UnitDelay  SampleTime=-1  HasFrameUpgradeWarning=on
  Output : Outport  VectorParamsAs1DForOutWhenUnconnected=off
  wires:
  TimeCount/1 -> CycleTrigger/2(In2)
  Condition/1 -> Switch3/2
  Constant8/1 -> Switch2/1
  CycleTrigger/1(Trigger) -> Switch2/2, Unit Delay3/1
  Constant10/1 -> Switch2/3
  Switch3/1 -> CycleTrigger/1(In1)
  Switch2/1 -> Unit Delay1/1
  Constant11/1 -> Switch3/3
  Unit Delay1/1 -> Switch3/1
  Unit Delay3/1 -> Output/1

== system EPT/Foreground_TimeBase_5ms/System Setup/Unit_Setup()/Delay3 ==
  Condition : Inport
  TimeCount : Inport  Port=2
  Constant10 : Constant
  Constant11 : Constant  Value=0
  Constant8 : Constant  Value=0
  CycleTrigger : Subsystem
  Switch2 : Switch  Threshold=1
  Switch3 : Switch  Threshold=1
  Unit Delay1 : UnitDelay  SampleTime=-1  HasFrameUpgradeWarning=on
  Unit Delay3 : UnitDelay  SampleTime=-1  HasFrameUpgradeWarning=on
  Output : Outport  VectorParamsAs1DForOutWhenUnconnected=off
  wires:
  TimeCount/1 -> CycleTrigger/2(In2)
  Condition/1 -> Switch3/2
  Constant8/1 -> Switch2/1
  CycleTrigger/1(Trigger) -> Switch2/2, Unit Delay3/1
  Constant10/1 -> Switch2/3
  Switch3/1 -> CycleTrigger/1(In1)
  Switch2/1 -> Unit Delay1/1
  Constant11/1 -> Switch3/3
  Unit Delay1/1 -> Switch3/1
  Unit Delay3/1 -> Output/1

== system EPT/Foreground_TimeBase_5ms/System Setup/Unit_Setup()/Delay4 ==
  Condition : Inport
  TimeCount : Inport  Port=2
  Constant10 : Constant
  Constant11 : Constant  Value=0
  Constant8 : Constant  Value=0
  CycleTrigger : Subsystem
  Switch2 : Switch  Threshold=1
  Switch3 : Switch  Threshold=1
  Unit Delay1 : UnitDelay  SampleTime=-1  HasFrameUpgradeWarning=on
  Unit Delay3 : UnitDelay  SampleTime=-1  HasFrameUpgradeWarning=on
  Output : Outport  VectorParamsAs1DForOutWhenUnconnected=off
  wires:
  Unit Delay3/1 -> Output/1
  Unit Delay1/1 -> Switch3/1
  Constant11/1 -> Switch3/3
  Switch2/1 -> Unit Delay1/1
  Switch3/1 -> CycleTrigger/1(In1)
  Constant10/1 -> Switch2/3
  CycleTrigger/1(Trigger) -> Unit Delay3/1, Switch2/2
  Constant8/1 -> Switch2/1
  Condition/1 -> Switch3/2
  TimeCount/1 -> CycleTrigger/2(In2)

== system EPT/Foreground_TimeBase_5ms/System Setup/Unit_Setup()/ECHS_CAN_Work ==
  Trigger : TriggerPort  VariantControl=Variant  PortDimensions=1
  Constant : Constant  OutDataTypeStr=boolean
  raptor_data_def5 : Raptor_lib/Data Storage/raptor_data_def  dataName='Flag_ECHS_CAN_Work'  initValue=0  dataType=boolean  storage=Volatile (RAM)  calVisible=on  calType=Measurement  calDispType=Number  calEnum={'False', 'True'}  calGain=1.0  calOffset=0  calMin=-inf  calMax=inf  calFormat='-1'  calUnit=''  calHelp=''  calAccess=1  calFunction=raptor_xcp_function(gcb)  calDispHeaders=off  calColHeaders={'Col1' 'Col2' 'Col3'}  calRowHeaders={'Row1' 'Row2' 'Row3'}
      settings: SourceProductName=Raptor
  raptor_data_write6 : Raptor_lib/Data Storage/raptor_data_write  dataName='Flag_ECHS_CAN_Work'  dataShape=Scalar  idxSource=Input Port  idxRow=1  idxCol=1
      settings: SourceProductName=Raptor
  wires:
  Constant/1 -> raptor_data_write6/1

== system EPT/Foreground_TimeBase_5ms/System Setup/Unit_Setup()/Relay_DCDC_12V_Off ==
  Trigger : TriggerPort  VariantControl=Variant  PortDimensions=1
  Constant : Constant  Value=0  OutDataTypeStr=boolean
  Data Type Conversion : DataTypeConversion
  NOT : Logic  Operator=NOT  IconShape=distinctive  AllPortsSameDT=off  OutDataTypeStr=boolean
  raptor_data_write1 : Raptor_lib/Data Storage/raptor_data_write  dataName='Relay_DCDC_12V'  dataShape=Scalar  idxSource=Input Port  idxRow=1  idxCol=1
      settings: SourceProductName=Raptor
  raptor_data_write2 : Raptor_lib/Data Storage/raptor_data_write  dataName='Cmd_DC_Control'  dataShape=Scalar  idxSource=Input Port  idxRow=1  idxCol=1
      settings: SourceProductName=Raptor
  wires:
  Constant/1 -> NOT/1, raptor_data_write1/1
  NOT/1 -> Data Type Conversion/1
  Data Type Conversion/1 -> raptor_data_write2/1

== system EPT/Foreground_TimeBase_5ms/System Setup/Unit_Setup()/Relay_DCDC_12V_On ==
  Trigger : TriggerPort  VariantControl=Variant  PortDimensions=1
  Constant : Constant  OutDataTypeStr=boolean
  Data Type Conversion : DataTypeConversion
  NOT : Logic  Operator=NOT  IconShape=distinctive  AllPortsSameDT=off  OutDataTypeStr=boolean
  raptor_data_write1 : Raptor_lib/Data Storage/raptor_data_write  dataName='Relay_DCDC_12V'  dataShape=Scalar  idxSource=Input Port  idxRow=1  idxCol=1
      settings: SourceProductName=Raptor
  raptor_data_write2 : Raptor_lib/Data Storage/raptor_data_write  dataName='Cmd_DC_Control'  dataShape=Scalar  idxSource=Input Port  idxRow=1  idxCol=1
      settings: SourceProductName=Raptor
  wires:
  Constant/1 -> NOT/1, raptor_data_write1/1
  NOT/1 -> Data Type Conversion/1
  Data Type Conversion/1 -> raptor_data_write2/1

== system EPT/Foreground_TimeBase_5ms/System Setup/Unit_Setup()/Relay_HV_Body_Off  ==
  Trigger : TriggerPort  VariantControl=Variant  PortDimensions=1
  Constant : Constant  Value=0  OutDataTypeStr=boolean
  raptor_data_write1 : Raptor_lib/Data Storage/raptor_data_write  dataName='Relay_HV_Body'  dataShape=Scalar  idxSource=Input Port  idxRow=1  idxCol=1
      settings: SourceProductName=Raptor
  wires:
  Constant/1 -> raptor_data_write1/1

== system EPT/Foreground_TimeBase_5ms/System Setup/Unit_Setup()/Relay_HV_Body_On  ==
  Trigger : TriggerPort  VariantControl=Variant  PortDimensions=1
  Constant : Constant  OutDataTypeStr=boolean
  raptor_data_write1 : Raptor_lib/Data Storage/raptor_data_write  dataName='Relay_HV_Body'  dataShape=Scalar  idxSource=Input Port  idxRow=1  idxCol=1
      settings: SourceProductName=Raptor
  wires:
  Constant/1 -> raptor_data_write1/1

== system EPT/I//O/Input/ADC_ChargerPlugInterface/Delay1 ==
  Condition : Inport
  TimeCount : Inport  Port=2
  Constant10 : Constant
  Constant11 : Constant  Value=0
  Constant8 : Constant  Value=0
  CycleTrigger : Subsystem
  Switch2 : Switch  Threshold=1
  Switch3 : Switch  Threshold=1
  Unit Delay1 : UnitDelay  SampleTime=-1  HasFrameUpgradeWarning=on
  Unit Delay2 : UnitDelay  SampleTime=-1  HasFrameUpgradeWarning=on
  Output : Outport  VectorParamsAs1DForOutWhenUnconnected=off
  wires:
  TimeCount/1 -> CycleTrigger/2(In2)
  Condition/1 -> Switch3/2
  CycleTrigger/1(Trigger) -> Switch2/2, Unit Delay1/1
  Constant8/1 -> Switch2/1
  Constant10/1 -> Switch2/3
  Switch3/1 -> CycleTrigger/1(In1)
  Constant11/1 -> Switch3/3
  Unit Delay2/1 -> Switch3/1
  Switch2/1 -> Unit Delay2/1
  Unit Delay1/1 -> Output/1

== system EPT/I//O/Input/ADC_ChargerPlugInterface/Delay2 ==
  Condition : Inport
  TimeCount : Inport  Port=2
  Constant10 : Constant
  Constant11 : Constant  Value=0
  Constant8 : Constant  Value=0
  CycleTrigger : Subsystem
  Switch2 : Switch  Threshold=1
  Switch3 : Switch  Threshold=1
  Unit Delay1 : UnitDelay  SampleTime=-1  HasFrameUpgradeWarning=on
  Unit Delay2 : UnitDelay  SampleTime=-1  HasFrameUpgradeWarning=on
  Output : Outport  VectorParamsAs1DForOutWhenUnconnected=off
  wires:
  Unit Delay1/1 -> Output/1
  Switch2/1 -> Unit Delay2/1
  Unit Delay2/1 -> Switch3/1
  Constant11/1 -> Switch3/3
  Switch3/1 -> CycleTrigger/1(In1)
  Constant10/1 -> Switch2/3
  Constant8/1 -> Switch2/1
  CycleTrigger/1(Trigger) -> Unit Delay1/1, Switch2/2
  Condition/1 -> Switch3/2
  TimeCount/1 -> CycleTrigger/2(In2)

== system EPT/I//O/Input/ADC_ChargerPlugInterface/Delay3 ==
  Condition : Inport
  TimeCount : Inport  Port=2
  Constant10 : Constant
  Constant11 : Constant  Value=0
  Constant8 : Constant  Value=0
  CycleTrigger : Subsystem
  Switch2 : Switch  Threshold=1
  Switch3 : Switch  Threshold=1
  Unit Delay1 : UnitDelay  SampleTime=-1  HasFrameUpgradeWarning=on
  Unit Delay2 : UnitDelay  SampleTime=-1  HasFrameUpgradeWarning=on
  Output : Outport  VectorParamsAs1DForOutWhenUnconnected=off
  wires:
  TimeCount/1 -> CycleTrigger/2(In2)
  Condition/1 -> Switch3/2
  CycleTrigger/1(Trigger) -> Switch2/2, Unit Delay1/1
  Constant8/1 -> Switch2/1
  Constant10/1 -> Switch2/3
  Switch3/1 -> CycleTrigger/1(In1)
  Constant11/1 -> Switch3/3
  Unit Delay2/1 -> Switch3/1
  Switch2/1 -> Unit Delay2/1
  Unit Delay1/1 -> Output/1

== system EPT/I//O/Input/ADC_ChargerPlugInterface/Latch1 ==
  Latch : Inport
  Reset : Inport  Port=2
  Switch1 : Switch  Criteria=u2 > Threshold
  Switch3 : Switch  Criteria=u2 > Threshold
  Unit Delay1 : UnitDelay  SampleTime=-1  HasFrameUpgradeWarning=on
  Output : Outport  VectorParamsAs1DForOutWhenUnconnected=off
  wires:
  Unit Delay1/1 -> Switch1/3
  Switch3/1 -> Output/1, Unit Delay1/1
  Reset/1 -> Switch3/2
  Latch/1 -> Switch1/1, Switch1/2
  Switch1/1 -> Switch3/3

== system EPT/I//O/Input/ADC_ChargerPlugInterface/Latch2 ==
  Latch : Inport
  Reset : Inport  Port=2
  Switch1 : Switch  Criteria=u2 > Threshold
  Switch3 : Switch  Criteria=u2 > Threshold
  Unit Delay1 : UnitDelay  SampleTime=-1  HasFrameUpgradeWarning=on
  Output : Outport  VectorParamsAs1DForOutWhenUnconnected=off
  wires:
  Switch1/1 -> Switch3/3
  Latch/1 -> Switch1/2, Switch1/1
  Reset/1 -> Switch3/2
  Switch3/1 -> Unit Delay1/1, Output/1
  Unit Delay1/1 -> Switch1/3

== system EPT/I//O/Input/ADC_ChargerPlugInterface/Latch3 ==
  Latch : Inport
  Reset : Inport  Port=2
  Switch1 : Switch  Criteria=u2 > Threshold
  Switch3 : Switch  Criteria=u2 > Threshold
  Unit Delay1 : UnitDelay  SampleTime=-1  HasFrameUpgradeWarning=on
  Output : Outport  VectorParamsAs1DForOutWhenUnconnected=off
  wires:
  Unit Delay1/1 -> Switch1/3
  Switch3/1 -> Output/1, Unit Delay1/1
  Reset/1 -> Switch3/2
  Latch/1 -> Switch1/1, Switch1/2
  Switch1/1 -> Switch3/3

== system EPT/LED_Status/DualLED_Funny/LED_Status/0.5Hz ==
  Trigger : TriggerPort  VariantControl=Variant  PortDimensions=1
  NOT : Logic  Operator=NOT  IconShape=distinctive  AllPortsSameDT=off  OutDataTypeStr=boolean
  raptor_data_def : Raptor_lib/Data Storage/raptor_data_def  dataName='Flag_LED_0_5Hz'  initValue=0  dataType=boolean  storage=Volatile (RAM)  calVisible=on  calType=Measurement  calDispType=Number  calEnum={'False', 'True'}  calGain=1.0  calOffset=0  calMin=-inf  calMax=inf  calFormat='-1'  calUnit=''  calHelp=''  calAccess=1  calFunction=raptor_xcp_function(gcb)  calDispHeaders=off  calColHeaders={'Col1' 'Col2' 'Col3'}  calRowHeaders={'Row1' 'Row2' 'Row3'}
      settings: SourceProductName=Raptor
  raptor_data_read : Raptor_lib/Data Storage/raptor_data_read  dataName='Flag_LED_0_5Hz'  dataShape=Scalar  idxSource=Input  idxRow=1  idxCol=1
      settings: SourceProductName=Raptor
  raptor_data_write1 : Raptor_lib/Data Storage/raptor_data_write  dataName='Flag_LED_0_5Hz'  dataShape=Scalar  idxSource=Input Port  idxRow=1  idxCol=1
      settings: SourceProductName=Raptor
  wires:
  NOT/1 -> raptor_data_write1/1
  raptor_data_read/1 -> NOT/1

== system EPT/LED_Status/DualLED_Funny/LED_Status/100Hz ==
  Trigger : TriggerPort  VariantControl=Variant  PortDimensions=1
  NOT : Logic  Operator=NOT  IconShape=distinctive  AllPortsSameDT=off  OutDataTypeStr=boolean
  raptor_data_def : Raptor_lib/Data Storage/raptor_data_def  dataName='Flag_LED_100Hz'  initValue=0  dataType=boolean  storage=Volatile (RAM)  calVisible=on  calType=Measurement  calDispType=Number  calEnum={'False', 'True'}  calGain=1.0  calOffset=0  calMin=-inf  calMax=inf  calFormat='-1'  calUnit=''  calHelp=''  calAccess=1  calFunction=raptor_xcp_function(gcb)  calDispHeaders=off  calColHeaders={'Col1' 'Col2' 'Col3'}  calRowHeaders={'Row1' 'Row2' 'Row3'}
      settings: SourceProductName=Raptor
  raptor_data_read : Raptor_lib/Data Storage/raptor_data_read  dataName='Flag_LED_100Hz'  dataShape=Scalar  idxSource=Input  idxRow=1  idxCol=1
      settings: SourceProductName=Raptor
  raptor_data_write1 : Raptor_lib/Data Storage/raptor_data_write  dataName='Flag_LED_100Hz'  dataShape=Scalar  idxSource=Input Port  idxRow=1  idxCol=1
      settings: SourceProductName=Raptor
  wires:
  raptor_data_read/1 -> NOT/1
  NOT/1 -> raptor_data_write1/1
